simulink model "mcb_pmsm_foc_sensorless_nucleo_f401re"  (R2024a)
settings: Solver=FixedStepDiscrete  StartTime=0.0  StopTime=inf  RelTol=1e-3  EnableMultiTasking=on
InitFcn:
  | stm32_pmsm_foc_data;
model workspace (MAT data in the model file):
  encoderResolution = 2000
  hallOffset = '0.5'
  indexOffset = 850
  polePairs = '4'
values from neighbouring files (symbols this model uses):
  acceleration = 20000/PU_System.N_base    [stm32_pmsm_foc_data.m]
  dataType = 'single'    [stm32_pmsm_foc_data.m]
  PI_params = mcb.internal.SetControllerParameters(pmsm,inverter,PU_System,T_pwm,2*Ts,Ts_speed)    [stm32_pmsm_foc_data.m]
  pmsm = mcb_SetPMSMMotorParameters('BLY172S')    [stm32_pmsm_foc_data.m]
  PU_System = mcb_SetPUSystem(pmsm,inverter)    [stm32_pmsm_foc_data.m]
  Speed_openLoop_PU = 0.1    [stm32_pmsm_foc_data.m]
  T_Ref_openLoop = 1    [stm32_pmsm_foc_data.m]
  Ts = T_pwm    (= 5e-05)    [stm32_pmsm_foc_data.m]
  Ts_motor = T_pwm/2    (= 2.5e-05)    [stm32_pmsm_foc_data.m]
  Ts_speed = 10*Ts    (= 0.0005)    [stm32_pmsm_foc_data.m]
undefined symbols (not defined in the file or in its folder): DiscIntNeverNeededParam, inverter, target
libraries: mcbcontrolslib x9, stm32f4xxblockslib x7, slpidlib x3, simulink x3, mcbsensorlessestimatorlib x1, mcbplantlib x1, mcbpositiondecoderlib x1, autolibpmsmexterior x1
(part 2 of 2)

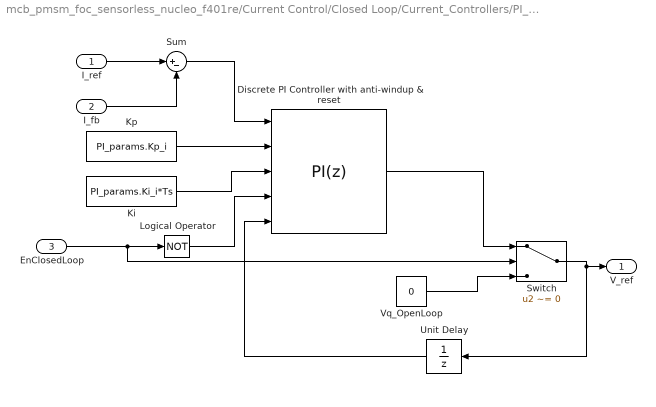
== system mcb_pmsm_foc_sensorless_nucleo_f401re/Current Control/Closed Loop/Current_Controllers/PI_Controller_Iq ==
  I_ref : Inport
  I_fb : Inport  Port=2
  EnClosedLoop : Inport  Port=3
  Discrete PI Controller with anti-windup & reset : slpidlib/PID Controller  Controller=PI  Form=Parallel  TimeDomain=Discrete-time  UseExternalTs=off  SampleTime=-1  IntegratorMethod=Forward Euler  FilterMethod=Forward Euler  ControllerParametersSource=external  P=1  I=1  UseKiTs=on  D=0  UseExternalDerivativeSource=off  N=100  UseFilter=on  TunerSelectOption=Transfer Function Based (PID Tuner App)  InitialConditionSource=external  InitialConditionForIntegrator=0  InitialConditionForFilter=0  DifferentiatorICPrevScaledInput=0  ExternalReset=level  TrackingMode=off  Kt=1  LimitOutput=on  SatLimitsSource=internal  UpperSaturationLimit=1  LowerSaturationLimit=-1  LinearizeAsGain=on  AntiWindupMode=clamping  Kb=1  LimitIntegrator=off  UpperIntegratorSaturationLimit=inf  LowerIntegratorSaturationLimit=-inf  RndMeth=Simplest  POutMin=[]  POutMax=[]  IOutMin=[]  IOutMax=[]  DOutMin=[]  DOutMax=[]  NOutMin=[]  NOutMax=[]  SumOutMin=[]  SumOutMax=[]  SaturationOutDataTypeStr=Inherit: Inherit via back propagation  SaturationOutMin=[]  SaturationOutMax=[]  PParamMin=[]  PParamMax=[]  IParamMin=[]  IParamMax=[]  DParamMin=[]  DParamMax=[]  NParamMin=[]  NParamMax=[]  KbParamMin=[]  KbParamMax=[]  KtParamMin=[]  KtParamMax=[]  KbOutMin=[]  KbOutMax=[]  KtOutMin=[]  KtOutMax=[]  IntegratorOutMin=[]  IntegratorOutMax=[]  FilterOutMin=[]  FilterOutMax=[]  SumI1OutMin=[]  SumI1OutMax=[]  SumI2OutMin=[]  SumI2OutMax=[]  SumI3OutMin=[]  SumI3OutMax=[]  SumI4OutMin=[]  SumI4OutMax=[]  SumDOutMin=[]  SumDOutMax=[]  DifferentiatorOutMin=[]  DifferentiatorOutMax=[]  FilterDiffOutCoefMin=[]  FilterDiffOutCoefMax=[]  ReciprocalOutMin=[]  ReciprocalOutMax=[]  SumDenOutMin=[]  SumDenOutMax=[]  SumNumOutMin=[]  SumNumOutMax=[]  DivideOutMin=[]  DivideOutMax=[]  UdiffTsProdOutMin=[]  UdiffTsProdOutMax=[]  NTsProdOutMin=[]  NTsProdOutMax=[]  UintegralTsProdOutMin=[]  UintegralTsProdOutMax=[]  UngainTsProdOutMin=[]  UngainTsProdOutMax=[]  ClampingZeroOutDataTypeStr=Inherit: Inherit via back propagation  ClampingZeroOutMin=[]  ClampingZeroOutMax=[]  FilterDenConstantOutDataTypeStr=Inherit: Inherit via back propagation  FilterDenConstantOutMin=[]  FilterDenConstantOutMax=[]  PCopyOutDataTypeStr=Inherit: Inherit via back propagation  PCopyOutMin=[]  PCopyOutMax=[]  NCopyOutDataTypeStr=Inherit: Inherit via back propagation  NCopyOutMin=[]  NCopyOutMax=[]  IntegratorContinuousStateAttributes=''  IntegratorStateMustResolveToSignalObject=off  IntegratorRTWStateStorageClass=Auto  FilterContinuousStateAttributes=''  FilterStateMustResolveToSignalObject=off  FilterRTWStateStorageClass=Auto  ParallelPVariant=ExternalParameters  IdealPVariant=Disabled  IVariant=ExternalParameters  DVariant=Disabled  IntegratorVariant=Discrete  SatVariant=Enabled  AWVariant=DiscClampingParallel  PCopyVariant=Disabled  TRVariant=Disabled  FdbkBlocksVariant=Forward  IdealPFdbkVariant=Disabled  SatFdbkVariant=Disabled  DerivativeFilterVariant=Disabled  NVariant=Disabled  NCopyVariant=Disabled_SignalSpec  FilterICVariant=Disabled  IntegratorICVariant=ExternalICs  ExternalResetVariant=ExternalReset  TRSumVariant=Passthrough  SumFdbkVariant=Disabled  SumVariant=Sum_PI  TsampFilterVariant=InternalTs  TsampNgainVariant=Passthrough  TsampIntegralVariant=Disabled_SignalSpec  ExternalSaturationOutDataTypeStr=Inherit: Same as second input  DerivativeSourceVariant=Disabled
      settings: LibrarySourceBlock=mcbcontrolslib/PI Controller
  Ki : Constant  Value=PI_params.Ki_i*Ts  OutDataTypeStr=dataType  SampleTime=-1
  Kp : Constant  Value=PI_params.Kp_i  OutDataTypeStr=dataType  SampleTime=-1
  Logical Operator : Logic  Operator=NOT  IconShape=distinctive  AllPortsSameDT=off  OutDataTypeStr=boolean
  Sum : Sum  Inputs=|+-  OutDataTypeStr=Inherit: Same as first input
  Switch : Switch  Criteria=u2 ~= 0  RndMeth=Simplest  SaturateOnIntegerOverflow=off  InputSameDT=off
  Unit Delay : UnitDelay  SampleTime=-1  HasFrameUpgradeWarning=on
  Vq_OpenLoop : Constant  Value=0  OutDataTypeStr=dataType  SampleTime=-1
  V_ref : Outport  VectorParamsAs1DForOutWhenUnconnected=off
  wires:
  Switch/1 -> V_ref/1, Unit Delay/1
  I_fb/1 -> Sum/2
  Sum/1 -> Discrete PI Controller with anti-windup & reset/1
  Kp/1 -> Discrete PI Controller with anti-windup & reset/2
  I_ref/1 -> Sum/1
  Ki/1 -> Discrete PI Controller with anti-windup & reset/3
  Logical Operator/1 -> Discrete PI Controller with anti-windup & reset/4
  Unit Delay/1 -> Discrete PI Controller with anti-windup & reset/5
  Discrete PI Controller with anti-windup & reset/1 -> Switch/1
  Vq_OpenLoop/1 -> Switch/3
  EnClosedLoop/1 -> Switch/2, Logical Operator/1

== system mcb_pmsm_foc_sensorless_nucleo_f401re/Current Control/Input Scaling/Calculate Phase Currents/Data_Type ==
  In1 : Inport
  Data_Type_Fixed_Point : Subsystem  VariantControl=~isequal(dataType,'single')
  Data_Type_Float : Subsystem  VariantControl=isequal(dataType,'single')
  Iab_meas_PU : Outport

== system mcb_pmsm_foc_sensorless_nucleo_f401re/Current Control/Input Scaling/Calculate position and speed/Sliding Mode Observer ==
  InputSignals : Inport
  Enable : Inport  Port=2
  Demux1 : Demux
  Logical Operator : Logic  Operator=NOT  IconShape=distinctive  AllPortsSameDT=off  OutDataTypeStr=boolean
  Mux : Mux  Inputs=2
  Sliding Mode Observer : mcbsensorlessestimatorlib/Sliding Mode Observer  InputUnit=Per-unit  BlkSampleTime=Ts  StatorResistance=pmsm.Rs + inverter.R_board  StatorInductance=pmsm.Ld  MaxApplicationSpeed=pmsm.N_base  PolePairs=pmsm.p  MaxStatorVoltage=PU_System.V_base  MaxStatorCurrent=PU_System.I_base  DisturbanceObserverGain=smo.BackEmfObsGain  CurrentObserverGain=smo.CurrentObsGain  CutoffFreq=smo.CutoffFreq  PositionUnit=Per unit  PositionDataType=dataType  SpeedUnit=Per unit  PerUnitSpeed=PU_System.N_base  SpeedDataType=dataType
  Position/Speed : Outport
  wires:
  Mux/1 -> Position/Speed/1
  Demux1/4 -> Sliding Mode Observer/4  "Ibeta"
  Demux1/3 -> Sliding Mode Observer/3  "Ialpha"
  Sliding Mode Observer/1 -> Mux/1
  InputSignals/1 -> Demux1/1
  Enable/1 -> Logical Operator/1
  Logical Operator/1 -> Sliding Mode Observer/5
  Sliding Mode Observer/2 -> Mux/2
  Demux1/1 -> Sliding Mode Observer/1
  Demux1/2 -> Sliding Mode Observer/2

== system mcb_pmsm_foc_sensorless_nucleo_f401re/Hardware Init/Offset Calculations/Codegen/Default ADC Offset ==
  Constant : Constant  Value=inverter.CtSensAOffset  OutDataTypeStr=Inherit: Inherit via back propagation
  Constant1 : Constant  Value=inverter.CtSensBOffset  OutDataTypeStr=Inherit: Inherit via back propagation
  Data Store Write1 : DataStoreWrite  DataStoreName=IaOffset  IndexOptions=Index vector (dialog)  Indices=1  OutputSizes=1
  Data Store Write2 : DataStoreWrite  DataStoreName=IbOffset  IndexOptions=Index vector (dialog)  Indices=1  OutputSizes=1
  IaOffset : Outport
  IbOffset : Outport  Port=2
  wires:
  Constant/1 -> IaOffset/1, Data Store Write1/1
  Constant1/1 -> IbOffset/1, Data Store Write2/1

== system mcb_pmsm_foc_sensorless_nucleo_f401re/Hardware Init/Offset Calculations/Simulation/Default ADC Offset ==
  Constant : Constant  Value=inverter.CtSensAOffset  OutDataTypeStr=Inherit: Inherit via back propagation
  Constant1 : Constant  Value=inverter.CtSensBOffset  OutDataTypeStr=Inherit: Inherit via back propagation
  Data Store Write1 : DataStoreWrite  DataStoreName=IaOffset  IndexOptions=Index vector (dialog)  Indices=1  OutputSizes=1
  Data Store Write2 : DataStoreWrite  DataStoreName=IbOffset  IndexOptions=Index vector (dialog)  Indices=1  OutputSizes=1
  IaOffset : Outport
  IbOffset : Outport  Port=2
  wires:
  Constant/1 -> IaOffset/1, Data Store Write1/1
  Constant1/1 -> IbOffset/1, Data Store Write2/1

== system mcb_pmsm_foc_sensorless_nucleo_f401re/Inverter and Motor - Plant Model/Simulation/Load_Profile (Torque)/Subsystem2 ==
  Initial Value : Inport
  Final Value : Inport  Port=2
  Enable Condition : Inport  Port=3
  Compare To Time : simulink/Logic and Bit Operations/Compare To Constant  relop=<=  const=time  OutDataTypeStr=boolean
  Integrate Time : DiscreteIntegrator  ExternalReset=rising  SampleTime=-1  SaturateOnIntegerOverflow=on  ICPrevOutput=DiscIntNeverNeededParam  ICPrevScaledInput=DiscIntNeverNeededParam
  Pass value : Switch  Criteria=u2 > Threshold  SaturateOnIntegerOverflow=off  InputSameDT=off
  Relational Operator : RelationalOperator  Operator=~=  OutDataTypeStr=boolean  RndMeth=Simplest  InputSameDT=off
  Time Step Increment : Constant
  Unit Delay : UnitDelay  SampleTime=-1  HasFrameUpgradeWarning=on
  Output : Outport
  wires:
  Time Step Increment/1 -> Integrate Time/1
  Compare To Time/1 -> Pass value/2
  Initial Value/1 -> Pass value/1
  Integrate Time/1 -> Compare To Time/1
  Final Value/1 -> Pass value/3
  Pass value/1 -> Output/1
  Relational Operator/1 -> Integrate Time/2
  Enable Condition/1 -> Unit Delay/1, Relational Operator/1
  Unit Delay/1 -> Relational Operator/2

== system mcb_pmsm_foc_sensorless_nucleo_f401re/Current Control/Input Scaling/Calculate Phase Currents/Data_Type/Data_Type_Fixed_Point ==
  In1 : Inport
  Data Type Conversion : DataTypeConversion  OutDataTypeStr=fixdt(1,32,17)  ConvertRealWorld=Stored Integer (SI)  RndMeth=Simplest  SaturateOnIntegerOverflow=off
  Data Type Conversion1 : DataTypeConversion  OutDataTypeStr=dataType  RndMeth=Simplest  SaturateOnIntegerOverflow=off
  Q17 per unit conversion : ArithShift  BitShiftNumber=-6
  Iab_meas_PU : Outport
  wires:
  In1/1 -> Q17 per unit conversion/1
  Data Type Conversion1/1 -> Iab_meas_PU/1
  Data Type Conversion/1 -> Data Type Conversion1/1
  Q17 per unit conversion/1 -> Data Type Conversion/1

== system mcb_pmsm_foc_sensorless_nucleo_f401re/Current Control/Input Scaling/Calculate Phase Currents/Data_Type/Data_Type_Float ==
  In1 : Inport
  Get ADC Voltage : Gain  Gain=target.ADC_Vref /target.ADC_MaxCount  OutDataTypeStr=dataType  RndMeth=Simplest
  Get Currents : Gain  Gain=1/inverter.ISenseVoltPerAmp  RndMeth=Simplest  OutDataTypeStr=Inherit: Same as input
  PU_Conversion : Gain  Gain=1/PU_System.I_base  RndMeth=Simplest  OutDataTypeStr=Inherit: Same as input
  Iab_meas_PU : Outport
  wires:
  Get ADC Voltage/1 -> Get Currents/1
  Get Currents/1 -> PU_Conversion/1
  PU_Conversion/1 -> Iab_meas_PU/1
  In1/1 -> Get ADC Voltage/1
